simulink model "ForwardConverter"  (R2018a)
settings: Solver=VariableStepAuto  StartTime=0.0  StopTime=0.1  RelTol=1e-3
libraries: powerlib x15, powerlib_meascontrol x4
settings Model: Creator=ozie  LastModifiedBy=ozie

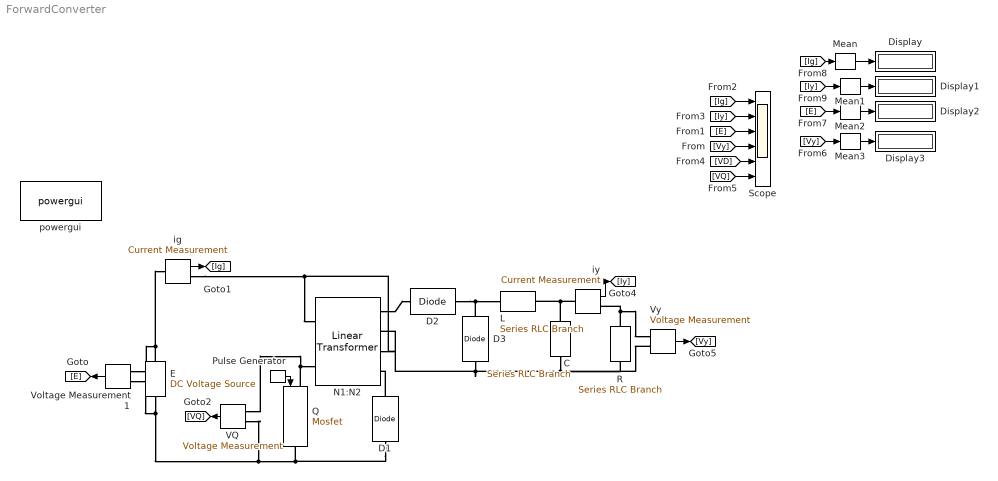
== system ForwardConverter ==
  C : powerlib/Elements/Series RLC Branch  LConnTagsString=__new0  RConnTagsString=__new0  BranchType=C  Resistance=1  Inductance=1e-3  SetiL0=off  InitialCurrent=0  Capacitance=100e-6  Setx0=off  InitialVoltage=0  Measurements=None
  D1 : powerlib/Power Electronics/Diode  Ron=0.001  Lon=0  Vf=0.8  IC=0  UseSnubber=0  Rs=500  Cs=250e-9  Measurements=off
  D2 : powerlib/Power Electronics/Diode  Ron=0.001  Lon=0  Vf=0.8  IC=0  UseSnubber=0  Rs=500  Cs=250e-9  Measurements=off
  D3 : powerlib/Power Electronics/Diode  Ron=0.001  Lon=0  Vf=0.8  IC=0  UseSnubber=0  Rs=500  Cs=250e-9  Measurements=off
  Display{,1..3} (4 alike) : Display
  E : powerlib/Electrical Sources/DC Voltage Source  Amplitude=100  Measurements=None
  L : powerlib/Elements/Series RLC Branch  LConnTagsString=__new0  RConnTagsString=__new0  BranchType=L  Resistance=0.8  Inductance=1e-3  SetiL0=off  InitialCurrent=0  Capacitance=1e-6  Setx0=off  InitialVoltage=0  Measurements=None
  Mean{,1..3} (4 alike) : powerlib_meascontrol/Measurements/Mean  Freq=60  Vinit=0  Ts=0
  N1:N2 : powerlib/Elements/Linear Transformer  UNITS=SI  NominalPower=[ 100 20000 ]  winding1="[100  0 0]"  winding2=[30 0 0]  ThreeWindings=on  winding3=[100 0 0]  RmLm=[1.0805e+06 2866]  Measurements=None  DataType=on
  Pulse Generator : DiscretePulseGenerator  PulseType=Time based  Period=1/20000  PulseWidth=50
  Q : powerlib/Power Electronics/Mosfet  Ron=0.1  Lon=0  Rd=0.01  Vfd=0  IC=0  Rs=1e5  Cs=inf  Measurements=off
  R : powerlib/Elements/Series RLC Branch  LConnTagsString=__new0  RConnTagsString=__new0  BranchType=R  Resistance=20  Inductance=1e-3  SetiL0=off  InitialCurrent=0  Capacitance=1e-6  Setx0=off  InitialVoltage=0  Measurements=None
  Scope : Scope  NumInputPorts=6
  VQ : powerlib/Measurements/Voltage Measurement  PhasorSimulation=off  OutputType=Complex  PSBequivalent=0
  Voltage Measurement1 : powerlib/Measurements/Voltage Measurement  PhasorSimulation=off  OutputType=Complex  PSBequivalent=0
  Vy : powerlib/Measurements/Voltage Measurement  PhasorSimulation=off  OutputType=Complex  PSBequivalent=0
  ig : powerlib/Measurements/Current Measurement  PhasorSimulation=off  OutputType=Complex  PSBequivalent=0
  iy : powerlib/Measurements/Current Measurement  PhasorSimulation=off  OutputType=Complex  PSBequivalent=0
  powergui : powerlib/powergui  Priority=1  SimulationMode=Continuous  SampleTime=50e-6  frequency=60  Iterations=50  frequencyindice=0  Pbase=100e6  ErrMax=1e-4  UnitsV=kV  UnitsW=MW  buscounter=0  FunctionMessages=off  echomessages=off  EnableUseOfTLC=off  CurrentSourceSwitches=off  DisableSnubberDevices=off  DisableRonSwitches=off  DisableVfSwitches=off  DisplayEquations=off  SolverType=Tustin/Backward Euler (TBE)  Interpol=off  ExternalGateDelay=off  methode=off  Ts=100  x0status=blocks  SPID=on  SwTol=0  HookPort=off  RestoreLinks=warning  ResistiveCurrentMeasurement=off  Frange=[0:2:500]  Ylog=off  Xlog=on  ShowGrid=off  save=off  variable=ZData  structure=0  ZoomFFT=off  StartTime=0.0  cycles=1  DisplayStyle=1  fundamental=60  FreqAxis=off  MaxFrequency=1000  frequencyindicesteady=1  RmsSteady=1  display=off
  wires:
  Mean/1 -> Display/1
  iy/1 -> [Iy]
  Mean3/1 -> Display3/1
  [Iy] -> Mean1/1
  Mean1/1 -> Display1/1
  [Vy] -> Mean3/1
  [VQ] -> Scope/6
  ig/1 -> [Ig]
  Pulse Generator/1 -> Q/1
  [Ig] -> Mean/1
  [Vy] -> Scope/4
  [VD] -> Scope/5
  [E] -> Scope/3
  Vy/1 -> [Vy]
  [E] -> Mean2/1
  Mean2/1 -> Display2/1
  [Ig] -> Scope/1
  VQ/1 -> [VQ]
  Voltage Measurement1/1 -> [E]
  [Iy] -> Scope/2
  connections:
  C/RConn1 -- Vy/LConn2 -- R/RConn1 -- D3/LConn1 -- N1:N2/RConn2
  VQ/LConn1 -- Q/LConn1 -- N1:N2/LConn2
  N1:N2/RConn1 -- D2/LConn1
  Voltage Measurement1/LConn1 -- ig/LConn1 -- E/RConn1
  D2/RConn1 -- L/LConn1 -- D3/RConn1
  Voltage Measurement1/LConn2 -- VQ/LConn2 -- D1/LConn1 -- Q/RConn1 -- E/LConn1
  R/LConn1 -- iy/RConn1 -- Vy/LConn1
  iy/LConn1 -- C/LConn1 -- L/RConn1
  ig/RConn1 -- N1:N2/RConn3 -- N1:N2/LConn1
  D1/RConn1 -- N1:N2/RConn4
